simulink model "EL_5MW_MVgrid_12pulse"  (R2025b)
settings: Solver=FixedStepDiscrete  StartTime=0.0  StopTime=1  FixedStep=5e-6  RelTol=1e-3
undefined symbols (not defined in the file): plecs
settings Model: Creator=ASUS  LastModifiedBy=ASUS

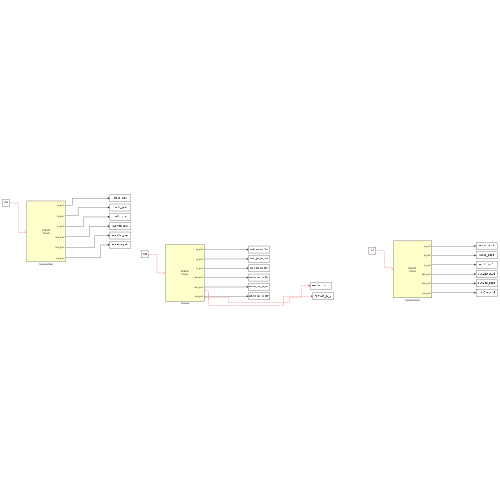
[thumbnail: Simulink's stored preview of the top-level diagram]
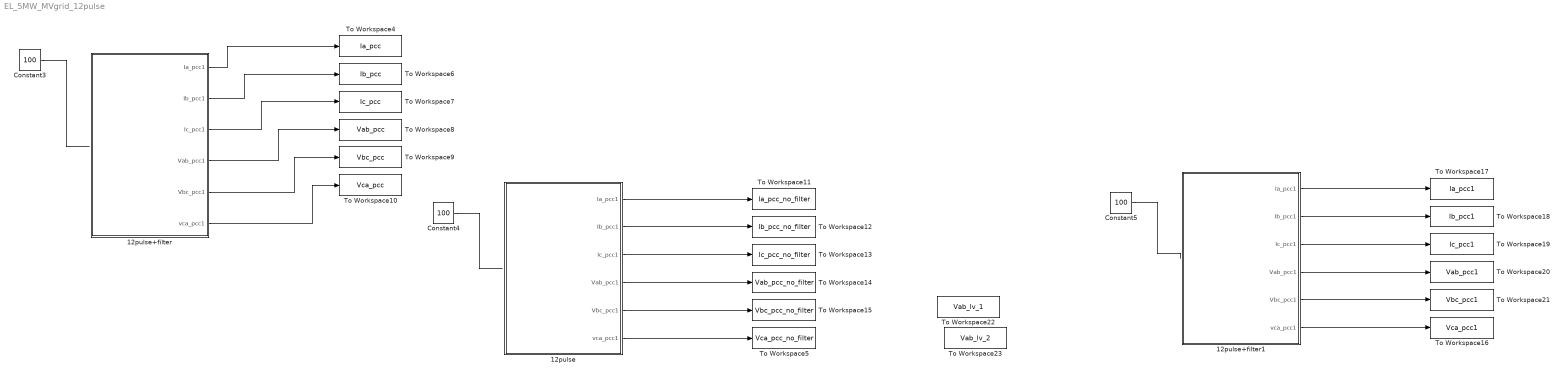
== system EL_5MW_MVgrid_12pulse ==
  12pulse : Subsystem  LoadFcn=plecs('sl', 200);  InitFcn=plecs('sl', 214);  StartFcn=plecs('sl', 208);  StopFcn=plecs('sl', 209);  mask(PlecsCircuit){PLECSData=<binary blob, 5368 chars, not shown>}
      mask prompts: PLECSData "PLECS Data (Do not delete or modify!)"
      mask init:
      | % PLACE CUSTOM INITIALIZATIONS ABOVE
      | % DO NOT REMOVE
      | plecs('sl', 215);
      | % DO NOT REMOVE
      settings: CopyFcn=plecs('sl', 203);  DeleteFcn=plecs('sl', 205);  UndoDeleteFcn=plecs('sl', 206);  PreSaveFcn=plecs('sl', 211);  PostSaveFcn=plecs('sl', 201);  NameChangeFcn=plecs('sl', 210);  DestroyFcn=plecs('sl', 207);  PreCopyFcn=plecs('sl', 216);  OpenFcn=plecs('sl', 202);  ErrorFcn=plerrorfcn
      mask Help: eval('plecs(''help'', ''qthelp:///creatingacircuit.html'')')
      mask Display: disp('PLECS\nCircuit')
  12pulse+filter : Subsystem  LoadFcn=plecs('sl', 200);  InitFcn=plecs('sl', 214);  StartFcn=plecs('sl', 208);  StopFcn=plecs('sl', 209);  mask(PlecsCircuit){PLECSData=<binary blob, 5784 chars, not shown>}
      mask prompts: PLECSData "PLECS Data (Do not delete or modify!)"
      mask init:
      | % PLACE CUSTOM INITIALIZATIONS ABOVE
      | % DO NOT REMOVE
      | plecs('sl', 215);
      | % DO NOT REMOVE
      settings: CopyFcn=plecs('sl', 203);  DeleteFcn=plecs('sl', 205);  UndoDeleteFcn=plecs('sl', 206);  PreSaveFcn=plecs('sl', 211);  PostSaveFcn=plecs('sl', 201);  NameChangeFcn=plecs('sl', 210);  DestroyFcn=plecs('sl', 207);  PreCopyFcn=plecs('sl', 216);  OpenFcn=plecs('sl', 202);  ErrorFcn=plerrorfcn
      mask Help: eval('plecs(''help'', ''qthelp:///creatingacircuit.html'')')
      mask Display: disp('PLECS\nCircuit')
  12pulse+filter1 : Subsystem  LoadFcn=plecs('sl', 200);  InitFcn=plecs('sl', 214);  StartFcn=plecs('sl', 208);  StopFcn=plecs('sl', 209);  mask(PlecsCircuit){PLECSData=<binary blob, 5364 chars, not shown>}
      mask prompts: PLECSData "PLECS Data (Do not delete or modify!)"
      mask init:
      | % PLACE CUSTOM INITIALIZATIONS ABOVE
      | % DO NOT REMOVE
      | plecs('sl', 215);
      | % DO NOT REMOVE
      settings: CopyFcn=plecs('sl', 203);  DeleteFcn=plecs('sl', 205);  UndoDeleteFcn=plecs('sl', 206);  PreSaveFcn=plecs('sl', 211);  PostSaveFcn=plecs('sl', 201);  NameChangeFcn=plecs('sl', 210);  DestroyFcn=plecs('sl', 207);  PreCopyFcn=plecs('sl', 216);  OpenFcn=plecs('sl', 202);  ErrorFcn=plerrorfcn
      mask Help: eval('plecs(''help'', ''qthelp:///creatingacircuit.html'')')
      mask Display: disp('PLECS\nCircuit')
  Constant3 : Constant  Value=100
  Constant4 : Constant  Value=100
  Constant5 : Constant  Value=100
  To Workspace10 : ToWorkspace  VariableName=Vca_pcc  SaveFormat=Structure With Time  SampleTime=-1
  To Workspace11 : ToWorkspace  VariableName=Ia_pcc_no_filter  SaveFormat=Structure With Time  SampleTime=-1
  To Workspace12 : ToWorkspace  VariableName=Ib_pcc_no_filter  SaveFormat=Structure With Time  SampleTime=-1
  To Workspace13 : ToWorkspace  VariableName=Ic_pcc_no_filter  SaveFormat=Structure With Time  SampleTime=-1
  To Workspace14 : ToWorkspace  VariableName=Vab_pcc_no_filter  SaveFormat=Structure With Time  SampleTime=-1
  To Workspace15 : ToWorkspace  VariableName=Vbc_pcc_no_filter  SaveFormat=Structure With Time  SampleTime=-1
  To Workspace16 : ToWorkspace  VariableName=Vca_pcc1  SaveFormat=Structure With Time  SampleTime=-1
  To Workspace17 : ToWorkspace  VariableName=Ia_pcc1  SaveFormat=Structure With Time  SampleTime=-1
  To Workspace18 : ToWorkspace  VariableName=Ib_pcc1  SaveFormat=Structure With Time  SampleTime=-1
  To Workspace19 : ToWorkspace  VariableName=Ic_pcc1  SaveFormat=Structure With Time  SampleTime=-1
  To Workspace20 : ToWorkspace  VariableName=Vab_pcc1  SaveFormat=Structure With Time  SampleTime=-1
  To Workspace21 : ToWorkspace  VariableName=Vbc_pcc1  SaveFormat=Structure With Time  SampleTime=-1
  To Workspace22 : ToWorkspace  VariableName=Vab_lv_1  SaveFormat=Timeseries  SampleTime=-1
  To Workspace23 : ToWorkspace  VariableName=Vab_lv_2  SaveFormat=Timeseries  SampleTime=-1
  To Workspace4 : ToWorkspace  VariableName=Ia_pcc  SaveFormat=Structure With Time  SampleTime=-1
  To Workspace5 : ToWorkspace  VariableName=Vca_pcc_no_filter  SaveFormat=Structure With Time  SampleTime=-1
  To Workspace6 : ToWorkspace  VariableName=Ib_pcc  SaveFormat=Structure With Time  SampleTime=-1
  To Workspace7 : ToWorkspace  VariableName=Ic_pcc  SaveFormat=Structure With Time  SampleTime=-1
  To Workspace8 : ToWorkspace  VariableName=Vab_pcc  SaveFormat=Structure With Time  SampleTime=-1
  To Workspace9 : ToWorkspace  VariableName=Vbc_pcc  SaveFormat=Structure With Time  SampleTime=-1
  wires:
  Constant3/1 -> ?
  12pulse+filter/1(Ia_pcc1) -> To Workspace4/1
  12pulse+filter/2(Ib_pcc1) -> To Workspace6/1
  12pulse+filter/3(Ic_pcc1) -> To Workspace7/1
  12pulse+filter/4(Vab_pcc1) -> To Workspace8/1
  12pulse+filter/5(Vbc_pcc1) -> To Workspace9/1
  12pulse+filter/6(vca_pcc1) -> To Workspace10/1
  12pulse/5(Vbc_pcc1) -> To Workspace15/1
  12pulse/3(Ic_pcc1) -> To Workspace13/1
  Constant4/1 -> ?
  12pulse/4(Vab_pcc1) -> To Workspace14/1
  12pulse/2(Ib_pcc1) -> To Workspace12/1
  12pulse/1(Ia_pcc1) -> To Workspace11/1
  12pulse/6(vca_pcc1) -> To Workspace5/1
  12pulse+filter1/5(Vbc_pcc1) -> To Workspace21/1
  12pulse+filter1/3(Ic_pcc1) -> To Workspace19/1
  Constant5/1 -> ?
  12pulse+filter1/4(Vab_pcc1) -> To Workspace20/1
  12pulse+filter1/2(Ib_pcc1) -> To Workspace18/1
  12pulse+filter1/1(Ia_pcc1) -> To Workspace17/1
  12pulse+filter1/6(vca_pcc1) -> To Workspace16/1
  ? -> To Workspace23/1
  ? -> To Workspace22/1

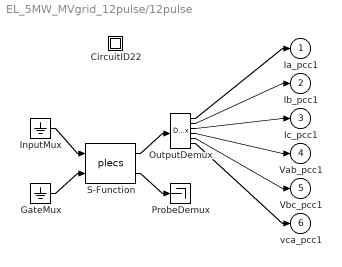
== system EL_5MW_MVgrid_12pulse/12pulse ==
  " CircuitID22 " : Subsystem
  " GateMux " : Ground
  " InputMux " : Ground
  " OutputDemux " : Demux  Outputs=[ 1 1 1 1 1 1 ]
  " ProbeDemux " : Terminator
  " S-Function " : S-Function  FunctionName=plecs  SFunctionDeploymentMode=off  EnableBusSupport=off
  Ia_pcc1 : Outport  PortDimensions=1
  Ib_pcc1 : Outport  Port=2  PortDimensions=1
  Ic_pcc1 : Outport  Port=3  PortDimensions=1
  Vab_pcc1 : Outport  Port=4  PortDimensions=1
  Vbc_pcc1 : Outport  Port=5  PortDimensions=1
  vca_pcc1 : Outport  Port=6  PortDimensions=1
  wires:
  " InputMux "/1 -> " S-Function "/1
  " GateMux "/1 -> " S-Function "/2
  " S-Function "/1 -> " OutputDemux "/1
  " S-Function "/2 -> " ProbeDemux "/1
  " OutputDemux "/1 -> Ia_pcc1/1
  " OutputDemux "/2 -> Ib_pcc1/1
  " OutputDemux "/3 -> Ic_pcc1/1
  " OutputDemux "/4 -> Vab_pcc1/1
  " OutputDemux "/5 -> Vbc_pcc1/1
  " OutputDemux "/6 -> vca_pcc1/1

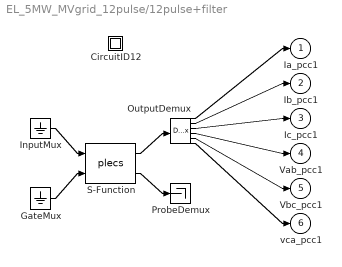
== system EL_5MW_MVgrid_12pulse/12pulse+filter ==
  " CircuitID12 " : Subsystem
  " GateMux " : Ground
  " InputMux " : Ground
  " OutputDemux " : Demux  Outputs=[ 1 1 1 1 1 1 ]
  " ProbeDemux " : Terminator
  " S-Function " : S-Function  FunctionName=plecs  SFunctionDeploymentMode=off  EnableBusSupport=off
  Ia_pcc1 : Outport  PortDimensions=1
  Ib_pcc1 : Outport  Port=2  PortDimensions=1
  Ic_pcc1 : Outport  Port=3  PortDimensions=1
  Vab_pcc1 : Outport  Port=4  PortDimensions=1
  Vbc_pcc1 : Outport  Port=5  PortDimensions=1
  vca_pcc1 : Outport  Port=6  PortDimensions=1
  wires:
  " InputMux "/1 -> " S-Function "/1
  " GateMux "/1 -> " S-Function "/2
  " S-Function "/1 -> " OutputDemux "/1
  " S-Function "/2 -> " ProbeDemux "/1
  " OutputDemux "/1 -> Ia_pcc1/1
  " OutputDemux "/2 -> Ib_pcc1/1
  " OutputDemux "/3 -> Ic_pcc1/1
  " OutputDemux "/4 -> Vab_pcc1/1
  " OutputDemux "/5 -> Vbc_pcc1/1
  " OutputDemux "/6 -> vca_pcc1/1

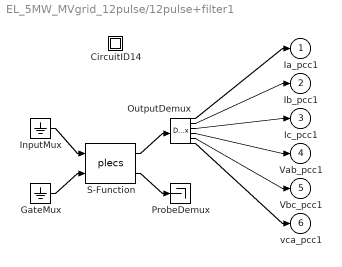
== system EL_5MW_MVgrid_12pulse/12pulse+filter1 ==
  " CircuitID14 " : Subsystem
  " GateMux " : Ground
  " InputMux " : Ground
  " OutputDemux " : Demux  Outputs=[ 1 1 1 1 1 1 ]
  " ProbeDemux " : Terminator
  " S-Function " : S-Function  FunctionName=plecs  SFunctionDeploymentMode=off  EnableBusSupport=off
  Ia_pcc1 : Outport  PortDimensions=1
  Ib_pcc1 : Outport  Port=2  PortDimensions=1
  Ic_pcc1 : Outport  Port=3  PortDimensions=1
  Vab_pcc1 : Outport  Port=4  PortDimensions=1
  Vbc_pcc1 : Outport  Port=5  PortDimensions=1
  vca_pcc1 : Outport  Port=6  PortDimensions=1
  wires:
  " InputMux "/1 -> " S-Function "/1
  " GateMux "/1 -> " S-Function "/2
  " S-Function "/1 -> " OutputDemux "/1
  " S-Function "/2 -> " ProbeDemux "/1
  " OutputDemux "/1 -> Ia_pcc1/1
  " OutputDemux "/2 -> Ib_pcc1/1
  " OutputDemux "/3 -> Ic_pcc1/1
  " OutputDemux "/4 -> Vab_pcc1/1
  " OutputDemux "/5 -> Vbc_pcc1/1
  " OutputDemux "/6 -> vca_pcc1/1

== system EL_5MW_MVgrid_12pulse/12pulse/ CircuitID22  ==

== system EL_5MW_MVgrid_12pulse/12pulse+filter/ CircuitID12  ==

== system EL_5MW_MVgrid_12pulse/12pulse+filter1/ CircuitID14  ==
